simulink model "manifold_matlab"  (R2018a)
settings: Solver=ode45  StartTime=0.0  StopTime=10.0  MaxStep=0.2  RelTol=1e-3  EnableMultiTasking=on
InitFcn:
  | load manifold_press_start.mat
settings Model: Creator=dlange  LastModifiedBy=bneiswan
settings DataIOCC: ExternalInput=[t, mdot_in, w]  LimitDataPoints=on  LoadExternalInput=on  SaveFormat=Array
settings OptimizationCC: ExpressionDepthLimit=2147483647  InitFltsAndDblsToZero=on  LifeSpan=inf
settings DebuggingCC: SaveWithParameterizedLinksMsg=none  UnderspecifiedInitializationDetection=Classic  MergeDetectMultiDrivingBlocksExec=none  SignalResolutionControl=TryResolveAllWithWarning  MultiTaskDSMMsg=warning  MultiTaskCondExecSysMsg=none  ParameterPrecisionLossMsg=none  FcnCallInpInsideContextMsg=warning  AllowSymbolicDim=off  StateNameClashWarn=warning  SFUnexpectedBacktrackingDiag=warning  SFNoUnconditionalDefaultTransitionDiag=warning  SFExecutionAtInitializationDiag=none
settings HardwareCC: ProdBitPerPointer=32  ProdBitPerSizeT=32  ProdBitPerPtrDiffT=32  ProdLargestAtomicFloat=None  ProdIntDivRoundTo=Undefined  ProdEndianess=Unspecified  ProdWordSize=32  ProdHWDeviceType=32-bit Generic
settings ModelReferenceCC: PropagateSignalLabelsOutOfModel=off
settings SFSimCC: SimParseCustomCode=off
settings CodeAppCC: StateflowObjectComments=on
settings GRTTargetCC: TargetFcnLib=ansi_tfl_tmw.mat  TargetLangStandard=C89/C90 (ANSI)  GeneratePreprocessorConditionals=Disable all  CombineOutputUpdateFcns=off  GRTInterface=on
settings ConfigComp: CovMetricSettings=dw  CovHtmlReporting=on  CovSaveCumulativeToWorkspaceVar=on  CovSaveSingleToWorkspaceVar=on  CovExternalEMLEnable=off  CovSFcnEnable=off

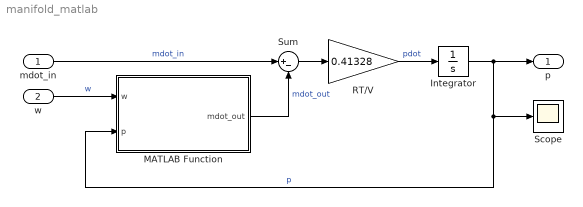
== system manifold_matlab ==
  mdot_in : Inport
  w : Inport  Port=2
  Integrator : Integrator  InitialCondition=0.543
      settings: AttributesFormatString=p0 = %<InitialCondition>
  MATLAB Function : MATLAB Function  TreatAsAtomicUnit=on
  RT/V : Gain  Gain=0.41328
  Scope : Scope
  Sum : Sum  Inputs=|+-
  p : Outport
  wires:
  Integrator/1 -> p/1, MATLAB Function/2(p), Scope/1  "p"
  RT/V/1 -> Integrator/1  "pdot"
  mdot_in/1 -> Sum/1  "mdot_in"
  Sum/1 -> RT/V/1
  w/1 -> MATLAB Function/1(w)  "w"
  MATLAB Function/1(mdot_out) -> Sum/2  "mdot_out"

== matlab function manifold_matlab/MATLAB Function ==
  data: w input; mdot_out output; p input
function mdot_out = mass_flow(w,p)
% This block uses MATLAB language features supported for
% code generation. See the help menu for details. 

mdot_out = -0.366 + 0.08979*w*p - 0.0337*w*p^2 + 0.0001*w^2*p;
